simulink model "correlator_core"  (Simulink 7.1)
settings: Solver=ode45  StartTime=0.0  StopTime=10000  RelTol=1e-3
libraries: xbsIndex_r4 x658, cfa_library x168, casper_library_delays x4, casper_library_misc x2
(part 3 of 9)

== system correlator_core/correlator_core/ctrl ==
  integ_time : Inport
  Logical : xbsIndex_r4/Logical  logical_function=AND  inputs=2  en=off  latency=0  precision=Full  arith_type=Unsigned  n_bits=16  bin_pt=0  align_bp=on  dbl_ovrd=off  block_type=logical
      settings: block_version=11.4
  Relational : xbsIndex_r4/Relational  mode=a=b  en=off  latency=1  dbl_ovrd=off  block_type=relational
  frame_cntr : xbsIndex_r4/Counter  cnt_type=Free Running  cnt_to=Inf  operation=Up  start_count=0  cnt_by_val=1  arith_type=Unsigned  n_bits=32  bin_pt=0  load_pin=off  rst=on  en=on  explicit_period=on  period=1  dbl_ovrd=off  use_behavioral_HDL=off  use_rpm=off  implementation=Fabric  block_type=counter
      settings: block_version=11.4
  integ_cntr : xbsIndex_r4/Counter  cnt_type=Free Running  cnt_to=Inf  operation=Up  start_count=0  cnt_by_val=1  arith_type=Unsigned  n_bits=32  bin_pt=0  load_pin=off  rst=off  en=on  explicit_period=on  period=1  dbl_ovrd=off  use_behavioral_HDL=off  use_rpm=off  implementation=Fabric  block_type=counter
      settings: block_version=11.4
  lag_cntr : xbsIndex_r4/Counter  cnt_type=Free Running  cnt_to=Inf  operation=Up  start_count=0  cnt_by_val=1  arith_type=Unsigned  n_bits=5  bin_pt=0  load_pin=off  rst=on  en=off  explicit_period=on  period=1  dbl_ovrd=off  use_behavioral_HDL=off  use_rpm=off  implementation=Fabric  block_type=counter
      settings: block_version=11.4
  posedge1 : casper_library_misc/posedge  Tag=Rising Edge Detector  SystemSampleTime=-1
  integs : Outport
  tag scope: frames=global, lags=global, new_acc=global
  wires:
  frame_cntr/1 -> Relational/2, [frames]
  Logical/1 -> frame_cntr/1
  Relational/1 -> posedge1/1
  posedge1/1 -> Logical/1, integ_cntr/1, [new_acc]
  integ_time/1 -> Relational/1
  integ_cntr/1 -> integs/1
  lag_cntr/1 -> [lags]
  [sync_out] -> Logical/2, lag_cntr/1
  [valid_out] -> frame_cntr/2

== system correlator_core/correlator_core/delay_wideband_prog ==
  sync : Inport
  delay : Inport  Port=2
  en : Inport  Port=3
  data_in1 : Inport  Port=4
  data_in2 : Inport  Port=5
  data_in3 : Inport  Port=6
  data_in4 : Inport  Port=7
  AddSub1 : xbsIndex_r4/AddSub  mode=Addition  use_carryin=off  use_carryout=off  en=off  latency=0  precision=Full  arith_type=Unsigned  n_bits=9  bin_pt=0  quantization=Truncate  overflow=Wrap  dbl_ovrd=off  use_behavioral_HDL=off  pipelined=off  use_rpm=on  hw_selection=Fabric  block_type=addsub
  AddSub2 : xbsIndex_r4/AddSub  mode=Addition  use_carryin=off  use_carryout=off  en=off  latency=0  precision=Full  arith_type=Unsigned  n_bits=9  bin_pt=0  quantization=Truncate  overflow=Wrap  dbl_ovrd=off  use_behavioral_HDL=off  pipelined=off  use_rpm=on  hw_selection=Fabric  block_type=addsub
  AddSub3 : xbsIndex_r4/AddSub  mode=Addition  use_carryin=off  use_carryout=off  en=off  latency=0  precision=Full  arith_type=Unsigned  n_bits=9  bin_pt=0  quantization=Truncate  overflow=Wrap  dbl_ovrd=off  use_behavioral_HDL=off  pipelined=off  use_rpm=on  hw_selection=Fabric  block_type=addsub
  Constant1 : xbsIndex_r4/Constant  arith_type=Unsigned  const=2  n_bits=2  bin_pt=0  explicit_period=on  period=1  equ=P=C  opselect=C  inp2=PCIN>>17  opr=+  inp1=P  carry=CIN  dbl_ovrd=off  block_type=constant
      settings: block_version=11.4
  Constant2 : xbsIndex_r4/Constant  arith_type=Unsigned  const=1  n_bits=2  bin_pt=0  explicit_period=on  period=1  equ=P=C  opselect=C  inp2=PCIN>>17  opr=+  inp1=P  carry=CIN  dbl_ovrd=off  block_type=constant
      settings: block_version=11.4
  Constant3 : xbsIndex_r4/Constant  arith_type=Unsigned  const=0  n_bits=2  bin_pt=0  explicit_period=on  period=1  equ=P=C  opselect=C  inp2=PCIN>>17  opr=+  inp1=P  carry=CIN  dbl_ovrd=off  block_type=constant
      settings: block_version=11.4
  Convert1 : xbsIndex_r4/Convert  arith_type=Unsigned  n_bits=1  bin_pt=0  quantization=Truncate  overflow=Wrap  latency=0  dbl_ovrd=off  pipeline=off  block_type=convert
      settings: block_version=11.4
  Convert2 : xbsIndex_r4/Convert  arith_type=Unsigned  n_bits=1  bin_pt=0  quantization=Truncate  overflow=Wrap  latency=0  dbl_ovrd=off  pipeline=off  block_type=convert
      settings: block_version=11.4
  Convert3 : xbsIndex_r4/Convert  arith_type=Unsigned  n_bits=1  bin_pt=0  quantization=Truncate  overflow=Wrap  latency=0  dbl_ovrd=off  pipeline=off  block_type=convert
      settings: block_version=11.4
  Relational1 : xbsIndex_r4/Relational  mode=a>b  en=off  latency=0  dbl_ovrd=off  block_type=relational
  Relational2 : xbsIndex_r4/Relational  mode=a>b  en=off  latency=0  dbl_ovrd=off  block_type=relational
  Relational3 : xbsIndex_r4/Relational  mode=a>b  en=off  latency=0  dbl_ovrd=off  block_type=relational
  barrel_switcher : Subsystem  AncestorBlock=casper_library_reorder/barrel_switcher  mask(barrel_switcher){n_inputs=2}
      mask prompts: n_inputs "Number of Inputs: (2^?)"
      mask help:
      | Shifts input to right by amount specified on sel,
      | wrapping around into higher order bits.
      mask init:
      | barrel_switcher_init(gcb,...
      |     'n_inputs', n_inputs);
      settings: AttributesFormatString=n_inputs=2
      mask Help: eval('xlWeb(''http://casper.berkeley.edu/wiki/Barrel_switcher'')')
  bram_rd_addrs : xbsIndex_r4/Slice  nbits=9  boolean_output=off  mode=Lower Bit Location + Width  bit1=0  base1=MSB of Input  bit0=2  base0=LSB of Input  dbl_ovrd=off  block_type=slice
  delay_dp : casper_library_delays/delay_bram_prog_dp  SystemSampleTime=-1  ram_bits=9  bram_latency=2
      link override wr_addr: cnt_type=Free Running  cnt_to=Inf  operation=Up  start_count=0  cnt_by_val=1  arith_type=Unsigned  n_bits=ram_bits  bin_pt=0  load_pin=off  rst=off  en=off  explicit_period=on  period=1  dbl_ovrd=off  use_behavioral_HDL=on  implementation=Fabric  use_rpm=on
      link override wr_addr: infoedit="Hardware notes: Free running counters are the least expensive in hardware.  A count limited counter is implemented by combining a counter with a comparator."  xl_area=[0, 0, 0, 0, 0, 0, 0]
  delay_dp1 : casper_library_delays/delay_bram_prog_dp  SystemSampleTime=-1  ram_bits=9  bram_latency=2
  delay_dp2 : casper_library_delays/delay_bram_prog_dp  SystemSampleTime=-1  ram_bits=9  bram_latency=2
  delay_dp3 : casper_library_delays/delay_bram_prog_dp  SystemSampleTime=-1  ram_bits=9  bram_latency=2
  delay_reg : xbsIndex_r4/Register  init=0  rst=off  en=on  dbl_ovrd=off  block_type=register
      settings: block_version=11.4
  delay_sel : xbsIndex_r4/Delay  en=off  latency=3  dbl_ovrd=off  reg_retiming=off  block_type=delay
      settings: block_version=11.4
  shift_sel : xbsIndex_r4/Slice  nbits=2  boolean_output=off  mode=Lower Bit Location + Width  bit1=0  base1=MSB of Input  bit0=0  base0=LSB of Input  dbl_ovrd=off  block_type=slice
  sync_delay : xbsIndex_r4/Delay  en=off  latency=3  dbl_ovrd=off  reg_retiming=off  block_type=delay
      settings: block_version=11.4
  sync_out : Outport
  data_out1 : Outport  Port=2
  data_out2 : Outport  Port=3
  data_out3 : Outport  Port=4
  data_out4 : Outport  Port=5
  wires:
  sync/1 -> sync_delay/1
  delay/1 -> delay_reg/1
  en/1 -> delay_reg/2
  delay_reg/1 -> bram_rd_addrs/1, shift_sel/1
  data_in1/1 -> delay_dp/1
  bram_rd_addrs/1 -> delay_dp/2, AddSub1/1, AddSub2/1, AddSub3/1
  sync_delay/1 -> barrel_switcher/2(sync_in)
  barrel_switcher/1(sync_out) -> sync_out/1
  barrel_switcher/5(Out4) -> data_out1/1
  delay_dp/1 -> barrel_switcher/6(In4)
  shift_sel/1 -> delay_sel/1, Relational1/1, Relational2/1, Relational3/1
  delay_sel/1 -> barrel_switcher/1(sel)
  Constant1/1 -> Relational1/2
  Relational1/1 -> Convert1/1
  Convert1/1 -> AddSub1/2
  AddSub1/1 -> delay_dp1/2
  data_in2/1 -> delay_dp1/1
  delay_dp1/1 -> barrel_switcher/5(In3)
  barrel_switcher/2(Out1) -> data_out4/1
  Constant2/1 -> Relational2/2
  Relational2/1 -> Convert2/1
  Convert2/1 -> AddSub2/2
  AddSub2/1 -> delay_dp2/2
  data_in3/1 -> delay_dp2/1
  delay_dp2/1 -> barrel_switcher/4(In2)
  barrel_switcher/3(Out2) -> data_out3/1
  Constant3/1 -> Relational3/2
  Relational3/1 -> Convert3/1
  Convert3/1 -> AddSub3/2
  AddSub3/1 -> delay_dp3/2
  data_in4/1 -> delay_dp3/1
  delay_dp3/1 -> barrel_switcher/3(In1)
  barrel_switcher/4(Out3) -> data_out2/1

== system correlator_core/correlator_core/simple_bram_vacc ==
  new_acc : Inport  OutDataType=sfix(16)  OutScaling=2^0
  din : Inport  Port=2  OutDataType=sfix(16)  OutScaling=2^0
  Adder : xbsIndex_r4/AddSub  mode=Addition  use_carryin=off  use_carryout=off  en=off  latency=add_latency  precision=User Defined  arith_type="Signed  (2's comp)"  n_bits=n_bits  bin_pt=bin_pt  quantization=Truncate  overflow=Wrap  dbl_ovrd=off  use_behavioral_HDL=off  pipelined=on  use_rpm=on  hw_selection=Fabric  block_type=addsub
      settings: xl_area=[0, 0, 0, 0, 0, 0, 0]  block_version=10.1.3
  Constant : xbsIndex_r4/Constant  arith_type=Signed (2's comp)  const=0  n_bits=n_bits  bin_pt=bin_pt  explicit_period=on  period=1  equ=P=C  opselect=C  inp2=PCIN>>17  opr=+  inp1=P  carry=CIN  dbl_ovrd=off  block_type=constant
  Mux : xbsIndex_r4/Mux  inputs=2  en=off  latency=0  precision=Full  arith_type="Signed  (2's comp)"  n_bits=8  bin_pt=2  quantization=Truncate  overflow=Wrap  dbl_ovrd=off  block_type=mux
      settings: xl_area=[0, 0, 0, 0, 0, 0, 0]
  delay_bram : Subsystem  mask(delay_bram){DelayLen=vec_len - add_latency, bram_latency=add_latency}
      mask prompts: DelayLen "Delay By:"; bram_latency "BRAM Latency"
      mask help: A delay block that uses BRAM for its storage.
      mask init:
      | if (DelayLen <= bram_latency)
      | 	error('delay value must be greater than BRAM Latency');
      | end
      | BitWidth = max(ceil(log2(DelayLen)), 2);
      mask Help: eval('xlWeb(''http://casper.berkeley.edu/wiki/Delay_bram'')')
  pulse_ext : Subsystem  mask(pulse_ext){pulse_len=vec_len}
      mask prompts: pulse_len "Length of Pulse"
      mask help:
      | Extends a boolean signal to be high for the specified number of clocks after
      | the last high input.
      mask init:
      | bits = ceil(log2(pulse_len+1));
      mask Help: eval('xlWeb(''http://casper.berkeley.edu/wiki/Pulse_ext'')')
  dout : Outport  OutDataType=sfix(16)  OutScaling=2^0
  valid : Outport  Port=2  OutDataType=sfix(16)  OutScaling=2^0
  wires:
  Adder/1 -> delay_bram/1(In1)
  delay_bram/1(Out1) -> dout/1, Mux/2
  new_acc/1 -> pulse_ext/1(in)
  din/1 -> Adder/1
  pulse_ext/1(out) -> Mux/1, valid/1
  Mux/1 -> Adder/2
  Constant/1 -> Mux/3

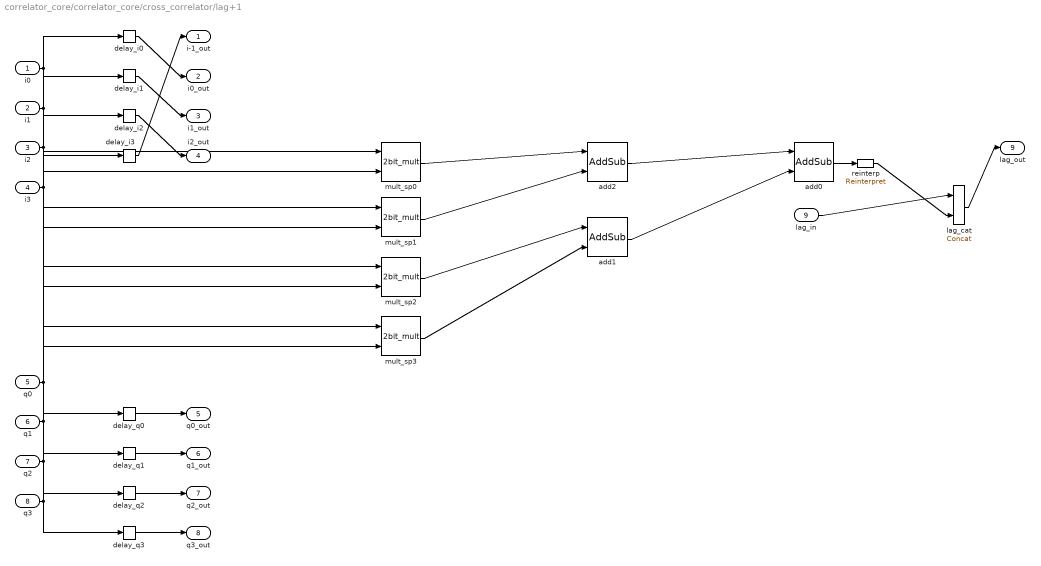
== system correlator_core/correlator_core/cross_correlator/lag+1 ==
  i0 : Inport
  i1 : Inport  Port=2
  i2 : Inport  Port=3
  i3 : Inport  Port=4
  q0 : Inport  Port=5
  q1 : Inport  Port=6
  q2 : Inport  Port=7
  q3 : Inport  Port=8
  lag_in : Inport  Port=9
  add0 : xbsIndex_r4/AddSub  mode=Addition  use_carryin=off  use_carryout=off  en=off  latency=2  precision=Full  arith_type=Unsigned  n_bits=16  bin_pt=14  quantization=Truncate  overflow=Wrap  dbl_ovrd=off  use_behavioral_HDL=on  pipelined=on  use_rpm=on  hw_selection=Fabric  block_type=addsub
  add1 : xbsIndex_r4/AddSub  mode=Addition  use_carryin=off  use_carryout=off  en=off  latency=2  precision=Full  arith_type=Unsigned  n_bits=16  bin_pt=14  quantization=Truncate  overflow=Wrap  dbl_ovrd=off  use_behavioral_HDL=on  pipelined=on  use_rpm=on  hw_selection=Fabric  block_type=addsub
      settings: block_version=10.1.3
  add2 : xbsIndex_r4/AddSub  mode=Addition  use_carryin=off  use_carryout=off  en=off  latency=2  precision=Full  arith_type=Unsigned  n_bits=16  bin_pt=14  quantization=Truncate  overflow=Wrap  dbl_ovrd=off  use_behavioral_HDL=on  pipelined=on  use_rpm=on  hw_selection=Fabric  block_type=addsub
      settings: block_version=10.1.3
  delay_i0 : xbsIndex_r4/Delay  en=off  latency=2  dbl_ovrd=off  reg_retiming=off  block_type=delay
      settings: block_version=11.4
  delay_i1 : xbsIndex_r4/Delay  en=off  latency=2  dbl_ovrd=off  reg_retiming=off  block_type=delay
      settings: block_version=11.4
  delay_i2 : xbsIndex_r4/Delay  en=off  latency=2  dbl_ovrd=off  reg_retiming=off  block_type=delay
  delay_i3 : xbsIndex_r4/Delay  en=off  latency=3  dbl_ovrd=off  reg_retiming=off  block_type=delay
  delay_q{0..3} (4 alike) : xbsIndex_r4/Delay  en=off  latency=2  dbl_ovrd=off  reg_retiming=off  block_type=delay
      delay_q0 settings: block_version=11.4
      delay_q1 settings: block_version=11.4
  lag_cat : xbsIndex_r4/Concat  num_inputs=2  dbl_ovrd=off  block_type=concat
  mult_sp{0..3} (4 alike) : cfa_library/2bit_mult  SystemSampleTime=-1
  reinterp : xbsIndex_r4/Reinterpret  force_arith_type=on  arith_type=Unsigned  force_bin_pt=on  bin_pt=0  block_type=reinterpret
      settings: infoedit="Changes signal type without altering the binary representation.   You can changed the signal between signed and unsigned, and relocate the binary point.<br><br>Hardware notes: In hardware this block costs nothing.<br><br>Example:  Suppose the input is 6 bits wide, signed, with 2 fractional bits, and the output is forced to unsigned with 0 fractional bits.  Then an input of -2.0 (1110.00 in binary 2's complement) becomes an output of 56 (111000 in binary)."
  i-1_out : Outport
  i0_out : Outport  Port=2
  i1_out : Outport  Port=3
  i2_out : Outport  Port=4
  q0_out : Outport  Port=5
  q1_out : Outport  Port=6
  q2_out : Outport  Port=7
  q3_out : Outport  Port=8
  lag_out : Outport  Port=9
  wires:
  i0/1 -> mult_sp0/1, delay_i0/1
  q0/1 -> mult_sp0/2, delay_q0/1
  i1/1 -> mult_sp1/1, delay_i1/1
  q1/1 -> mult_sp1/2, delay_q1/1
  i2/1 -> mult_sp2/1, delay_i2/1
  q2/1 -> mult_sp2/2, delay_q2/1
  i3/1 -> mult_sp3/1, delay_i3/1
  q3/1 -> mult_sp3/2, delay_q3/1
  mult_sp0/1 -> add2/1
  mult_sp1/1 -> add2/2
  mult_sp2/1 -> add1/1
  mult_sp3/1 -> add1/2
  add2/1 -> add0/1
  add1/1 -> add0/2
  delay_i0/1 -> i0_out/1
  delay_q0/1 -> q0_out/1
  delay_i1/1 -> i1_out/1
  delay_q1/1 -> q1_out/1
  delay_i2/1 -> i2_out/1
  delay_q2/1 -> q2_out/1
  delay_i3/1 -> i-1_out/1
  delay_q3/1 -> q3_out/1
  lag_in/1 -> lag_cat/1
  add0/1 -> reinterp/1
  reinterp/1 -> lag_cat/2
  lag_cat/1 -> lag_out/1

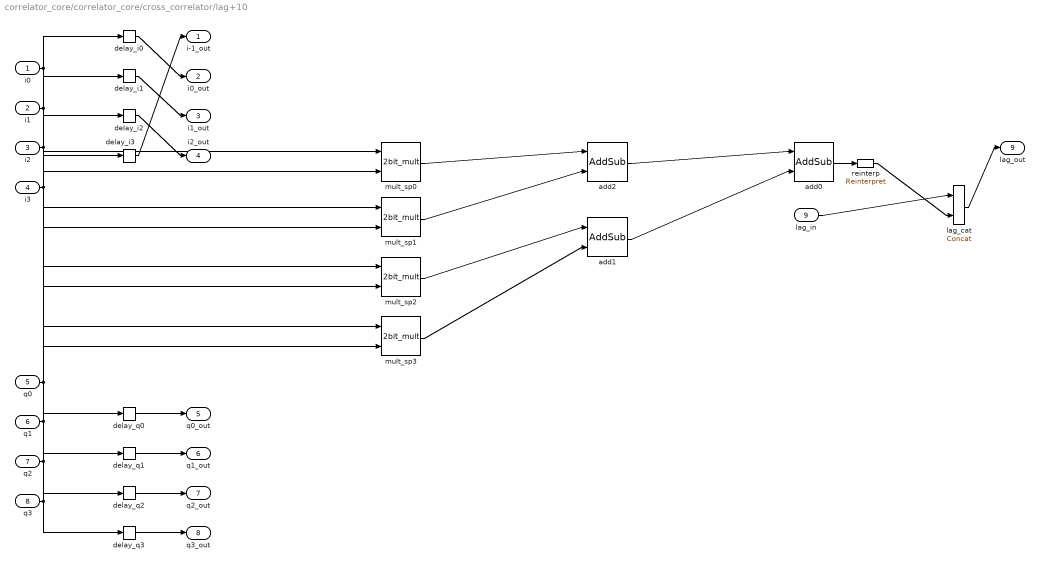
== system correlator_core/correlator_core/cross_correlator/lag+10 ==
  i0 : Inport
  i1 : Inport  Port=2
  i2 : Inport  Port=3
  i3 : Inport  Port=4
  q0 : Inport  Port=5
  q1 : Inport  Port=6
  q2 : Inport  Port=7
  q3 : Inport  Port=8
  lag_in : Inport  Port=9
  add0 : xbsIndex_r4/AddSub  mode=Addition  use_carryin=off  use_carryout=off  en=off  latency=2  precision=Full  arith_type=Unsigned  n_bits=16  bin_pt=14  quantization=Truncate  overflow=Wrap  dbl_ovrd=off  use_behavioral_HDL=on  pipelined=on  use_rpm=on  hw_selection=Fabric  block_type=addsub
  add1 : xbsIndex_r4/AddSub  mode=Addition  use_carryin=off  use_carryout=off  en=off  latency=2  precision=Full  arith_type=Unsigned  n_bits=16  bin_pt=14  quantization=Truncate  overflow=Wrap  dbl_ovrd=off  use_behavioral_HDL=on  pipelined=on  use_rpm=on  hw_selection=Fabric  block_type=addsub
      settings: block_version=10.1.3
  add2 : xbsIndex_r4/AddSub  mode=Addition  use_carryin=off  use_carryout=off  en=off  latency=2  precision=Full  arith_type=Unsigned  n_bits=16  bin_pt=14  quantization=Truncate  overflow=Wrap  dbl_ovrd=off  use_behavioral_HDL=on  pipelined=on  use_rpm=on  hw_selection=Fabric  block_type=addsub
      settings: block_version=10.1.3
  delay_i0 : xbsIndex_r4/Delay  en=off  latency=2  dbl_ovrd=off  reg_retiming=off  block_type=delay
      settings: block_version=11.4
  delay_i1 : xbsIndex_r4/Delay  en=off  latency=2  dbl_ovrd=off  reg_retiming=off  block_type=delay
      settings: block_version=11.4
  delay_i2 : xbsIndex_r4/Delay  en=off  latency=2  dbl_ovrd=off  reg_retiming=off  block_type=delay
  delay_i3 : xbsIndex_r4/Delay  en=off  latency=3  dbl_ovrd=off  reg_retiming=off  block_type=delay
  delay_q{0..3} (4 alike) : xbsIndex_r4/Delay  en=off  latency=2  dbl_ovrd=off  reg_retiming=off  block_type=delay
      delay_q0 settings: block_version=11.4
      delay_q1 settings: block_version=11.4
  lag_cat : xbsIndex_r4/Concat  num_inputs=2  dbl_ovrd=off  block_type=concat
  mult_sp{0..3} (4 alike) : cfa_library/2bit_mult  SystemSampleTime=-1
  reinterp : xbsIndex_r4/Reinterpret  force_arith_type=on  arith_type=Unsigned  force_bin_pt=on  bin_pt=0  block_type=reinterpret
      settings: infoedit="Changes signal type without altering the binary representation.   You can changed the signal between signed and unsigned, and relocate the binary point.<br><br>Hardware notes: In hardware this block costs nothing.<br><br>Example:  Suppose the input is 6 bits wide, signed, with 2 fractional bits, and the output is forced to unsigned with 0 fractional bits.  Then an input of -2.0 (1110.00 in binary 2's complement) becomes an output of 56 (111000 in binary)."
  i-1_out : Outport
  i0_out : Outport  Port=2
  i1_out : Outport  Port=3
  i2_out : Outport  Port=4
  q0_out : Outport  Port=5
  q1_out : Outport  Port=6
  q2_out : Outport  Port=7
  q3_out : Outport  Port=8
  lag_out : Outport  Port=9
  wires:
  i0/1 -> mult_sp0/1, delay_i0/1
  q0/1 -> mult_sp0/2, delay_q0/1
  i1/1 -> mult_sp1/1, delay_i1/1
  q1/1 -> mult_sp1/2, delay_q1/1
  i2/1 -> mult_sp2/1, delay_i2/1
  q2/1 -> mult_sp2/2, delay_q2/1
  i3/1 -> mult_sp3/1, delay_i3/1
  q3/1 -> mult_sp3/2, delay_q3/1
  mult_sp0/1 -> add2/1
  mult_sp1/1 -> add2/2
  mult_sp2/1 -> add1/1
  mult_sp3/1 -> add1/2
  add2/1 -> add0/1
  add1/1 -> add0/2
  delay_i0/1 -> i0_out/1
  delay_q0/1 -> q0_out/1
  delay_i1/1 -> i1_out/1
  delay_q1/1 -> q1_out/1
  delay_i2/1 -> i2_out/1
  delay_q2/1 -> q2_out/1
  delay_i3/1 -> i-1_out/1
  delay_q3/1 -> q3_out/1
  lag_in/1 -> lag_cat/1
  add0/1 -> reinterp/1
  reinterp/1 -> lag_cat/2
  lag_cat/1 -> lag_out/1

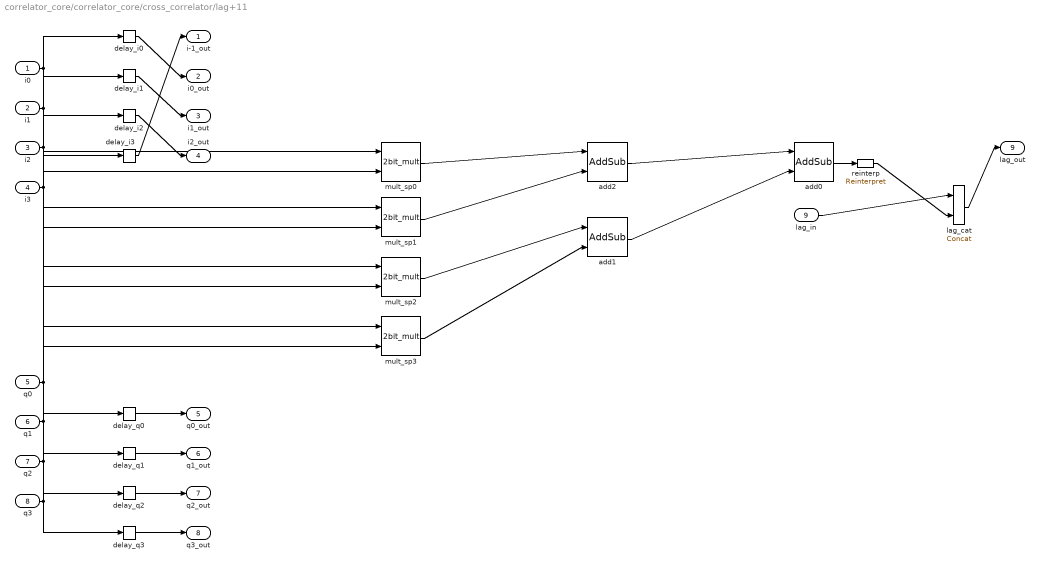
== system correlator_core/correlator_core/cross_correlator/lag+11 ==
  i0 : Inport
  i1 : Inport  Port=2
  i2 : Inport  Port=3
  i3 : Inport  Port=4
  q0 : Inport  Port=5
  q1 : Inport  Port=6
  q2 : Inport  Port=7
  q3 : Inport  Port=8
  lag_in : Inport  Port=9
  add0 : xbsIndex_r4/AddSub  mode=Addition  use_carryin=off  use_carryout=off  en=off  latency=2  precision=Full  arith_type=Unsigned  n_bits=16  bin_pt=14  quantization=Truncate  overflow=Wrap  dbl_ovrd=off  use_behavioral_HDL=on  pipelined=on  use_rpm=on  hw_selection=Fabric  block_type=addsub
  add1 : xbsIndex_r4/AddSub  mode=Addition  use_carryin=off  use_carryout=off  en=off  latency=2  precision=Full  arith_type=Unsigned  n_bits=16  bin_pt=14  quantization=Truncate  overflow=Wrap  dbl_ovrd=off  use_behavioral_HDL=on  pipelined=on  use_rpm=on  hw_selection=Fabric  block_type=addsub
      settings: block_version=10.1.3
  add2 : xbsIndex_r4/AddSub  mode=Addition  use_carryin=off  use_carryout=off  en=off  latency=2  precision=Full  arith_type=Unsigned  n_bits=16  bin_pt=14  quantization=Truncate  overflow=Wrap  dbl_ovrd=off  use_behavioral_HDL=on  pipelined=on  use_rpm=on  hw_selection=Fabric  block_type=addsub
      settings: block_version=10.1.3
  delay_i0 : xbsIndex_r4/Delay  en=off  latency=2  dbl_ovrd=off  reg_retiming=off  block_type=delay
      settings: block_version=11.4
  delay_i1 : xbsIndex_r4/Delay  en=off  latency=2  dbl_ovrd=off  reg_retiming=off  block_type=delay
      settings: block_version=11.4
  delay_i2 : xbsIndex_r4/Delay  en=off  latency=2  dbl_ovrd=off  reg_retiming=off  block_type=delay
  delay_i3 : xbsIndex_r4/Delay  en=off  latency=3  dbl_ovrd=off  reg_retiming=off  block_type=delay
  delay_q{0..3} (4 alike) : xbsIndex_r4/Delay  en=off  latency=2  dbl_ovrd=off  reg_retiming=off  block_type=delay
      delay_q0 settings: block_version=11.4
      delay_q1 settings: block_version=11.4
  lag_cat : xbsIndex_r4/Concat  num_inputs=2  dbl_ovrd=off  block_type=concat
  mult_sp{0..3} (4 alike) : cfa_library/2bit_mult  SystemSampleTime=-1
  reinterp : xbsIndex_r4/Reinterpret  force_arith_type=on  arith_type=Unsigned  force_bin_pt=on  bin_pt=0  block_type=reinterpret
      settings: infoedit="Changes signal type without altering the binary representation.   You can changed the signal between signed and unsigned, and relocate the binary point.<br><br>Hardware notes: In hardware this block costs nothing.<br><br>Example:  Suppose the input is 6 bits wide, signed, with 2 fractional bits, and the output is forced to unsigned with 0 fractional bits.  Then an input of -2.0 (1110.00 in binary 2's complement) becomes an output of 56 (111000 in binary)."
  i-1_out : Outport
  i0_out : Outport  Port=2
  i1_out : Outport  Port=3
  i2_out : Outport  Port=4
  q0_out : Outport  Port=5
  q1_out : Outport  Port=6
  q2_out : Outport  Port=7
  q3_out : Outport  Port=8
  lag_out : Outport  Port=9
  wires:
  i0/1 -> mult_sp0/1, delay_i0/1
  q0/1 -> mult_sp0/2, delay_q0/1
  i1/1 -> mult_sp1/1, delay_i1/1
  q1/1 -> mult_sp1/2, delay_q1/1
  i2/1 -> mult_sp2/1, delay_i2/1
  q2/1 -> mult_sp2/2, delay_q2/1
  i3/1 -> mult_sp3/1, delay_i3/1
  q3/1 -> mult_sp3/2, delay_q3/1
  mult_sp0/1 -> add2/1
  mult_sp1/1 -> add2/2
  mult_sp2/1 -> add1/1
  mult_sp3/1 -> add1/2
  add2/1 -> add0/1
  add1/1 -> add0/2
  delay_i0/1 -> i0_out/1
  delay_q0/1 -> q0_out/1
  delay_i1/1 -> i1_out/1
  delay_q1/1 -> q1_out/1
  delay_i2/1 -> i2_out/1
  delay_q2/1 -> q2_out/1
  delay_i3/1 -> i-1_out/1
  delay_q3/1 -> q3_out/1
  lag_in/1 -> lag_cat/1
  add0/1 -> reinterp/1
  reinterp/1 -> lag_cat/2
  lag_cat/1 -> lag_out/1

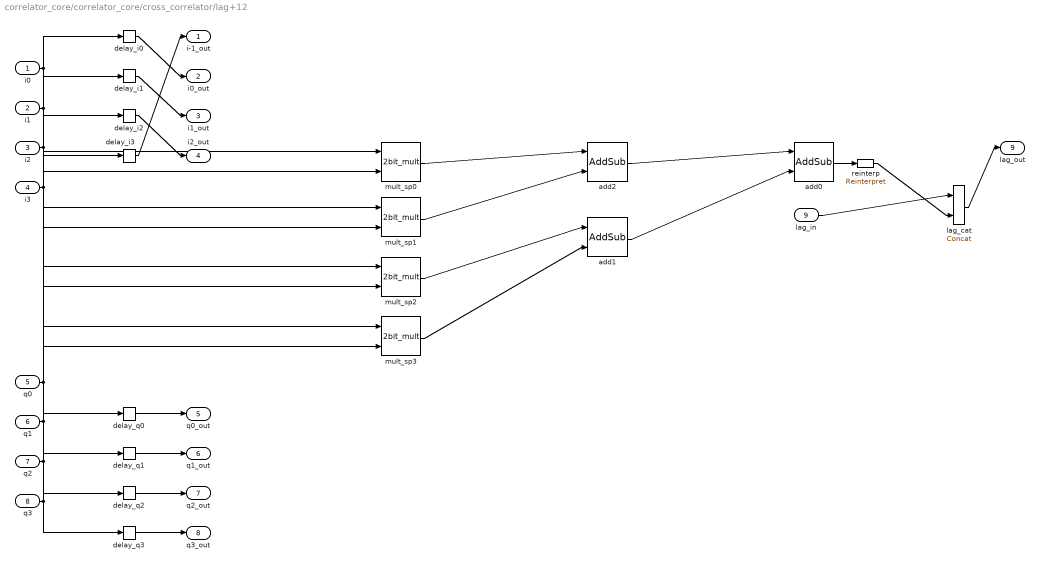
== system correlator_core/correlator_core/cross_correlator/lag+12 ==
  i0 : Inport
  i1 : Inport  Port=2
  i2 : Inport  Port=3
  i3 : Inport  Port=4
  q0 : Inport  Port=5
  q1 : Inport  Port=6
  q2 : Inport  Port=7
  q3 : Inport  Port=8
  lag_in : Inport  Port=9
  add0 : xbsIndex_r4/AddSub  mode=Addition  use_carryin=off  use_carryout=off  en=off  latency=2  precision=Full  arith_type=Unsigned  n_bits=16  bin_pt=14  quantization=Truncate  overflow=Wrap  dbl_ovrd=off  use_behavioral_HDL=on  pipelined=on  use_rpm=on  hw_selection=Fabric  block_type=addsub
  add1 : xbsIndex_r4/AddSub  mode=Addition  use_carryin=off  use_carryout=off  en=off  latency=2  precision=Full  arith_type=Unsigned  n_bits=16  bin_pt=14  quantization=Truncate  overflow=Wrap  dbl_ovrd=off  use_behavioral_HDL=on  pipelined=on  use_rpm=on  hw_selection=Fabric  block_type=addsub
      settings: block_version=10.1.3
  add2 : xbsIndex_r4/AddSub  mode=Addition  use_carryin=off  use_carryout=off  en=off  latency=2  precision=Full  arith_type=Unsigned  n_bits=16  bin_pt=14  quantization=Truncate  overflow=Wrap  dbl_ovrd=off  use_behavioral_HDL=on  pipelined=on  use_rpm=on  hw_selection=Fabric  block_type=addsub
      settings: block_version=10.1.3
  delay_i0 : xbsIndex_r4/Delay  en=off  latency=2  dbl_ovrd=off  reg_retiming=off  block_type=delay
      settings: block_version=11.4
  delay_i1 : xbsIndex_r4/Delay  en=off  latency=2  dbl_ovrd=off  reg_retiming=off  block_type=delay
      settings: block_version=11.4
  delay_i2 : xbsIndex_r4/Delay  en=off  latency=2  dbl_ovrd=off  reg_retiming=off  block_type=delay
  delay_i3 : xbsIndex_r4/Delay  en=off  latency=3  dbl_ovrd=off  reg_retiming=off  block_type=delay
  delay_q{0..3} (4 alike) : xbsIndex_r4/Delay  en=off  latency=2  dbl_ovrd=off  reg_retiming=off  block_type=delay
      delay_q0 settings: block_version=11.4
      delay_q1 settings: block_version=11.4
  lag_cat : xbsIndex_r4/Concat  num_inputs=2  dbl_ovrd=off  block_type=concat
  mult_sp{0..3} (4 alike) : cfa_library/2bit_mult  SystemSampleTime=-1
  reinterp : xbsIndex_r4/Reinterpret  force_arith_type=on  arith_type=Unsigned  force_bin_pt=on  bin_pt=0  block_type=reinterpret
      settings: infoedit="Changes signal type without altering the binary representation.   You can changed the signal between signed and unsigned, and relocate the binary point.<br><br>Hardware notes: In hardware this block costs nothing.<br><br>Example:  Suppose the input is 6 bits wide, signed, with 2 fractional bits, and the output is forced to unsigned with 0 fractional bits.  Then an input of -2.0 (1110.00 in binary 2's complement) becomes an output of 56 (111000 in binary)."
  i-1_out : Outport
  i0_out : Outport  Port=2
  i1_out : Outport  Port=3
  i2_out : Outport  Port=4
  q0_out : Outport  Port=5
  q1_out : Outport  Port=6
  q2_out : Outport  Port=7
  q3_out : Outport  Port=8
  lag_out : Outport  Port=9
  wires:
  i0/1 -> mult_sp0/1, delay_i0/1
  q0/1 -> mult_sp0/2, delay_q0/1
  i1/1 -> mult_sp1/1, delay_i1/1
  q1/1 -> mult_sp1/2, delay_q1/1
  i2/1 -> mult_sp2/1, delay_i2/1
  q2/1 -> mult_sp2/2, delay_q2/1
  i3/1 -> mult_sp3/1, delay_i3/1
  q3/1 -> mult_sp3/2, delay_q3/1
  mult_sp0/1 -> add2/1
  mult_sp1/1 -> add2/2
  mult_sp2/1 -> add1/1
  mult_sp3/1 -> add1/2
  add2/1 -> add0/1
  add1/1 -> add0/2
  delay_i0/1 -> i0_out/1
  delay_q0/1 -> q0_out/1
  delay_i1/1 -> i1_out/1
  delay_q1/1 -> q1_out/1
  delay_i2/1 -> i2_out/1
  delay_q2/1 -> q2_out/1
  delay_i3/1 -> i-1_out/1
  delay_q3/1 -> q3_out/1
  lag_in/1 -> lag_cat/1
  add0/1 -> reinterp/1
  reinterp/1 -> lag_cat/2
  lag_cat/1 -> lag_out/1

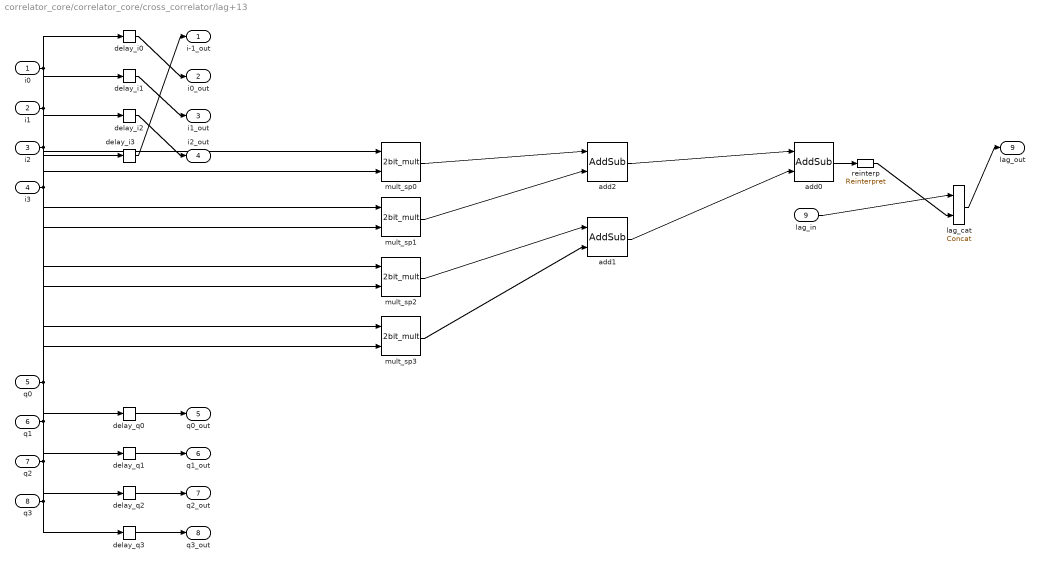
== system correlator_core/correlator_core/cross_correlator/lag+13 ==
  i0 : Inport
  i1 : Inport  Port=2
  i2 : Inport  Port=3
  i3 : Inport  Port=4
  q0 : Inport  Port=5
  q1 : Inport  Port=6
  q2 : Inport  Port=7
  q3 : Inport  Port=8
  lag_in : Inport  Port=9
  add0 : xbsIndex_r4/AddSub  mode=Addition  use_carryin=off  use_carryout=off  en=off  latency=2  precision=Full  arith_type=Unsigned  n_bits=16  bin_pt=14  quantization=Truncate  overflow=Wrap  dbl_ovrd=off  use_behavioral_HDL=on  pipelined=on  use_rpm=on  hw_selection=Fabric  block_type=addsub
  add1 : xbsIndex_r4/AddSub  mode=Addition  use_carryin=off  use_carryout=off  en=off  latency=2  precision=Full  arith_type=Unsigned  n_bits=16  bin_pt=14  quantization=Truncate  overflow=Wrap  dbl_ovrd=off  use_behavioral_HDL=on  pipelined=on  use_rpm=on  hw_selection=Fabric  block_type=addsub
      settings: block_version=10.1.3
  add2 : xbsIndex_r4/AddSub  mode=Addition  use_carryin=off  use_carryout=off  en=off  latency=2  precision=Full  arith_type=Unsigned  n_bits=16  bin_pt=14  quantization=Truncate  overflow=Wrap  dbl_ovrd=off  use_behavioral_HDL=on  pipelined=on  use_rpm=on  hw_selection=Fabric  block_type=addsub
      settings: block_version=10.1.3
  delay_i0 : xbsIndex_r4/Delay  en=off  latency=2  dbl_ovrd=off  reg_retiming=off  block_type=delay
      settings: block_version=11.4
  delay_i1 : xbsIndex_r4/Delay  en=off  latency=2  dbl_ovrd=off  reg_retiming=off  block_type=delay
      settings: block_version=11.4
  delay_i2 : xbsIndex_r4/Delay  en=off  latency=2  dbl_ovrd=off  reg_retiming=off  block_type=delay
  delay_i3 : xbsIndex_r4/Delay  en=off  latency=3  dbl_ovrd=off  reg_retiming=off  block_type=delay
  delay_q{0..3} (4 alike) : xbsIndex_r4/Delay  en=off  latency=2  dbl_ovrd=off  reg_retiming=off  block_type=delay
      delay_q0 settings: block_version=11.4
      delay_q1 settings: block_version=11.4
  lag_cat : xbsIndex_r4/Concat  num_inputs=2  dbl_ovrd=off  block_type=concat
  mult_sp{0..3} (4 alike) : cfa_library/2bit_mult  SystemSampleTime=-1
  reinterp : xbsIndex_r4/Reinterpret  force_arith_type=on  arith_type=Unsigned  force_bin_pt=on  bin_pt=0  block_type=reinterpret
      settings: infoedit="Changes signal type without altering the binary representation.   You can changed the signal between signed and unsigned, and relocate the binary point.<br><br>Hardware notes: In hardware this block costs nothing.<br><br>Example:  Suppose the input is 6 bits wide, signed, with 2 fractional bits, and the output is forced to unsigned with 0 fractional bits.  Then an input of -2.0 (1110.00 in binary 2's complement) becomes an output of 56 (111000 in binary)."
  i-1_out : Outport
  i0_out : Outport  Port=2
  i1_out : Outport  Port=3
  i2_out : Outport  Port=4
  q0_out : Outport  Port=5
  q1_out : Outport  Port=6
  q2_out : Outport  Port=7
  q3_out : Outport  Port=8
  lag_out : Outport  Port=9
  wires:
  i0/1 -> mult_sp0/1, delay_i0/1
  q0/1 -> mult_sp0/2, delay_q0/1
  i1/1 -> mult_sp1/1, delay_i1/1
  q1/1 -> mult_sp1/2, delay_q1/1
  i2/1 -> mult_sp2/1, delay_i2/1
  q2/1 -> mult_sp2/2, delay_q2/1
  i3/1 -> mult_sp3/1, delay_i3/1
  q3/1 -> mult_sp3/2, delay_q3/1
  mult_sp0/1 -> add2/1
  mult_sp1/1 -> add2/2
  mult_sp2/1 -> add1/1
  mult_sp3/1 -> add1/2
  add2/1 -> add0/1
  add1/1 -> add0/2
  delay_i0/1 -> i0_out/1
  delay_q0/1 -> q0_out/1
  delay_i1/1 -> i1_out/1
  delay_q1/1 -> q1_out/1
  delay_i2/1 -> i2_out/1
  delay_q2/1 -> q2_out/1
  delay_i3/1 -> i-1_out/1
  delay_q3/1 -> q3_out/1
  lag_in/1 -> lag_cat/1
  add0/1 -> reinterp/1
  reinterp/1 -> lag_cat/2
  lag_cat/1 -> lag_out/1

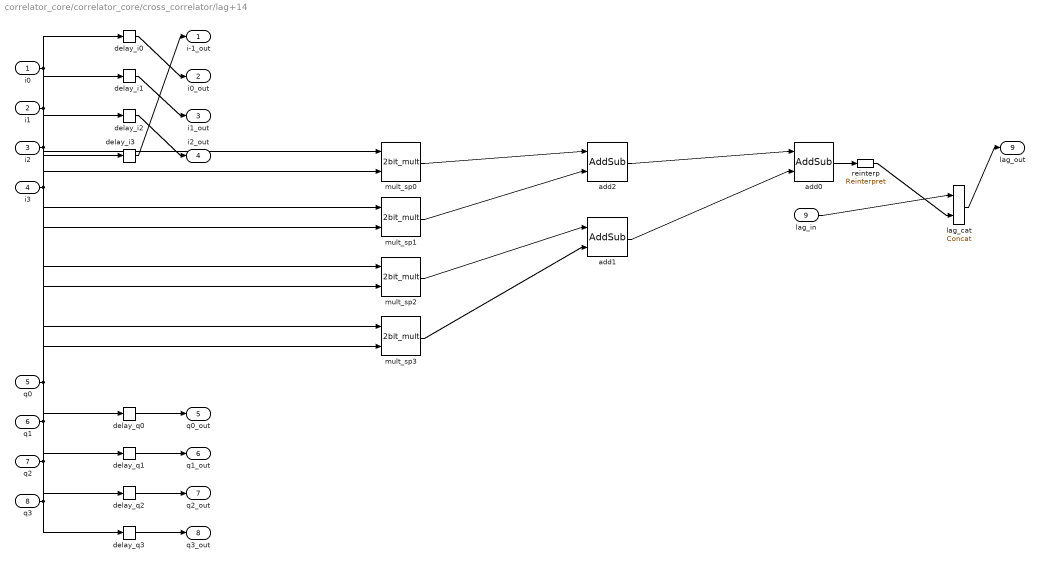
== system correlator_core/correlator_core/cross_correlator/lag+14 ==
  i0 : Inport
  i1 : Inport  Port=2
  i2 : Inport  Port=3
  i3 : Inport  Port=4
  q0 : Inport  Port=5
  q1 : Inport  Port=6
  q2 : Inport  Port=7
  q3 : Inport  Port=8
  lag_in : Inport  Port=9
  add0 : xbsIndex_r4/AddSub  mode=Addition  use_carryin=off  use_carryout=off  en=off  latency=2  precision=Full  arith_type=Unsigned  n_bits=16  bin_pt=14  quantization=Truncate  overflow=Wrap  dbl_ovrd=off  use_behavioral_HDL=on  pipelined=on  use_rpm=on  hw_selection=Fabric  block_type=addsub
  add1 : xbsIndex_r4/AddSub  mode=Addition  use_carryin=off  use_carryout=off  en=off  latency=2  precision=Full  arith_type=Unsigned  n_bits=16  bin_pt=14  quantization=Truncate  overflow=Wrap  dbl_ovrd=off  use_behavioral_HDL=on  pipelined=on  use_rpm=on  hw_selection=Fabric  block_type=addsub
      settings: block_version=10.1.3
  add2 : xbsIndex_r4/AddSub  mode=Addition  use_carryin=off  use_carryout=off  en=off  latency=2  precision=Full  arith_type=Unsigned  n_bits=16  bin_pt=14  quantization=Truncate  overflow=Wrap  dbl_ovrd=off  use_behavioral_HDL=on  pipelined=on  use_rpm=on  hw_selection=Fabric  block_type=addsub
      settings: block_version=10.1.3
  delay_i0 : xbsIndex_r4/Delay  en=off  latency=2  dbl_ovrd=off  reg_retiming=off  block_type=delay
      settings: block_version=11.4
  delay_i1 : xbsIndex_r4/Delay  en=off  latency=2  dbl_ovrd=off  reg_retiming=off  block_type=delay
      settings: block_version=11.4
  delay_i2 : xbsIndex_r4/Delay  en=off  latency=2  dbl_ovrd=off  reg_retiming=off  block_type=delay
  delay_i3 : xbsIndex_r4/Delay  en=off  latency=3  dbl_ovrd=off  reg_retiming=off  block_type=delay
  delay_q{0..3} (4 alike) : xbsIndex_r4/Delay  en=off  latency=2  dbl_ovrd=off  reg_retiming=off  block_type=delay
      delay_q0 settings: block_version=11.4
      delay_q1 settings: block_version=11.4
  lag_cat : xbsIndex_r4/Concat  num_inputs=2  dbl_ovrd=off  block_type=concat
  mult_sp{0..3} (4 alike) : cfa_library/2bit_mult  SystemSampleTime=-1
  reinterp : xbsIndex_r4/Reinterpret  force_arith_type=on  arith_type=Unsigned  force_bin_pt=on  bin_pt=0  block_type=reinterpret
      settings: infoedit="Changes signal type without altering the binary representation.   You can changed the signal between signed and unsigned, and relocate the binary point.<br><br>Hardware notes: In hardware this block costs nothing.<br><br>Example:  Suppose the input is 6 bits wide, signed, with 2 fractional bits, and the output is forced to unsigned with 0 fractional bits.  Then an input of -2.0 (1110.00 in binary 2's complement) becomes an output of 56 (111000 in binary)."
  i-1_out : Outport
  i0_out : Outport  Port=2
  i1_out : Outport  Port=3
  i2_out : Outport  Port=4
  q0_out : Outport  Port=5
  q1_out : Outport  Port=6
  q2_out : Outport  Port=7
  q3_out : Outport  Port=8
  lag_out : Outport  Port=9
  wires:
  i0/1 -> mult_sp0/1, delay_i0/1
  q0/1 -> mult_sp0/2, delay_q0/1
  i1/1 -> mult_sp1/1, delay_i1/1
  q1/1 -> mult_sp1/2, delay_q1/1
  i2/1 -> mult_sp2/1, delay_i2/1
  q2/1 -> mult_sp2/2, delay_q2/1
  i3/1 -> mult_sp3/1, delay_i3/1
  q3/1 -> mult_sp3/2, delay_q3/1
  mult_sp0/1 -> add2/1
  mult_sp1/1 -> add2/2
  mult_sp2/1 -> add1/1
  mult_sp3/1 -> add1/2
  add2/1 -> add0/1
  add1/1 -> add0/2
  delay_i0/1 -> i0_out/1
  delay_q0/1 -> q0_out/1
  delay_i1/1 -> i1_out/1
  delay_q1/1 -> q1_out/1
  delay_i2/1 -> i2_out/1
  delay_q2/1 -> q2_out/1
  delay_i3/1 -> i-1_out/1
  delay_q3/1 -> q3_out/1
  lag_in/1 -> lag_cat/1
  add0/1 -> reinterp/1
  reinterp/1 -> lag_cat/2
  lag_cat/1 -> lag_out/1

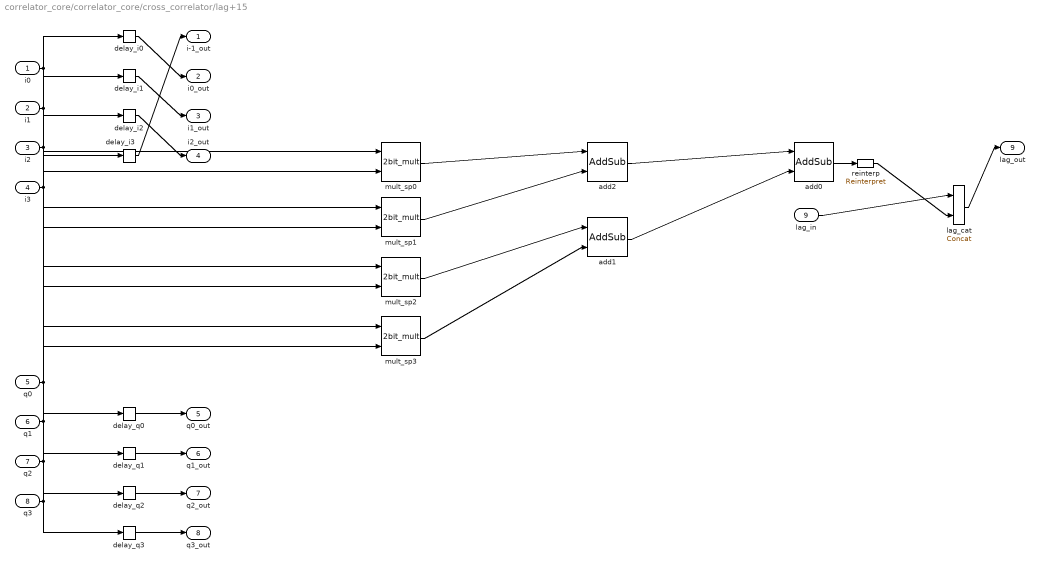
== system correlator_core/correlator_core/cross_correlator/lag+15 ==
  i0 : Inport
  i1 : Inport  Port=2
  i2 : Inport  Port=3
  i3 : Inport  Port=4
  q0 : Inport  Port=5
  q1 : Inport  Port=6
  q2 : Inport  Port=7
  q3 : Inport  Port=8
  lag_in : Inport  Port=9
  add0 : xbsIndex_r4/AddSub  mode=Addition  use_carryin=off  use_carryout=off  en=off  latency=2  precision=Full  arith_type=Unsigned  n_bits=16  bin_pt=14  quantization=Truncate  overflow=Wrap  dbl_ovrd=off  use_behavioral_HDL=on  pipelined=on  use_rpm=on  hw_selection=Fabric  block_type=addsub
  add1 : xbsIndex_r4/AddSub  mode=Addition  use_carryin=off  use_carryout=off  en=off  latency=2  precision=Full  arith_type=Unsigned  n_bits=16  bin_pt=14  quantization=Truncate  overflow=Wrap  dbl_ovrd=off  use_behavioral_HDL=on  pipelined=on  use_rpm=on  hw_selection=Fabric  block_type=addsub
      settings: block_version=10.1.3
  add2 : xbsIndex_r4/AddSub  mode=Addition  use_carryin=off  use_carryout=off  en=off  latency=2  precision=Full  arith_type=Unsigned  n_bits=16  bin_pt=14  quantization=Truncate  overflow=Wrap  dbl_ovrd=off  use_behavioral_HDL=on  pipelined=on  use_rpm=on  hw_selection=Fabric  block_type=addsub
      settings: block_version=10.1.3
  delay_i0 : xbsIndex_r4/Delay  en=off  latency=2  dbl_ovrd=off  reg_retiming=off  block_type=delay
      settings: block_version=11.4
  delay_i1 : xbsIndex_r4/Delay  en=off  latency=2  dbl_ovrd=off  reg_retiming=off  block_type=delay
      settings: block_version=11.4
  delay_i2 : xbsIndex_r4/Delay  en=off  latency=2  dbl_ovrd=off  reg_retiming=off  block_type=delay
  delay_i3 : xbsIndex_r4/Delay  en=off  latency=3  dbl_ovrd=off  reg_retiming=off  block_type=delay
  delay_q{0..3} (4 alike) : xbsIndex_r4/Delay  en=off  latency=2  dbl_ovrd=off  reg_retiming=off  block_type=delay
      delay_q0 settings: block_version=11.4
      delay_q1 settings: block_version=11.4
  lag_cat : xbsIndex_r4/Concat  num_inputs=2  dbl_ovrd=off  block_type=concat
  mult_sp{0..3} (4 alike) : cfa_library/2bit_mult  SystemSampleTime=-1
  reinterp : xbsIndex_r4/Reinterpret  force_arith_type=on  arith_type=Unsigned  force_bin_pt=on  bin_pt=0  block_type=reinterpret
      settings: infoedit="Changes signal type without altering the binary representation.   You can changed the signal between signed and unsigned, and relocate the binary point.<br><br>Hardware notes: In hardware this block costs nothing.<br><br>Example:  Suppose the input is 6 bits wide, signed, with 2 fractional bits, and the output is forced to unsigned with 0 fractional bits.  Then an input of -2.0 (1110.00 in binary 2's complement) becomes an output of 56 (111000 in binary)."
  i-1_out : Outport
  i0_out : Outport  Port=2
  i1_out : Outport  Port=3
  i2_out : Outport  Port=4
  q0_out : Outport  Port=5
  q1_out : Outport  Port=6
  q2_out : Outport  Port=7
  q3_out : Outport  Port=8
  lag_out : Outport  Port=9
  wires:
  i0/1 -> mult_sp0/1, delay_i0/1
  q0/1 -> mult_sp0/2, delay_q0/1
  i1/1 -> mult_sp1/1, delay_i1/1
  q1/1 -> mult_sp1/2, delay_q1/1
  i2/1 -> mult_sp2/1, delay_i2/1
  q2/1 -> mult_sp2/2, delay_q2/1
  i3/1 -> mult_sp3/1, delay_i3/1
  q3/1 -> mult_sp3/2, delay_q3/1
  mult_sp0/1 -> add2/1
  mult_sp1/1 -> add2/2
  mult_sp2/1 -> add1/1
  mult_sp3/1 -> add1/2
  add2/1 -> add0/1
  add1/1 -> add0/2
  delay_i0/1 -> i0_out/1
  delay_q0/1 -> q0_out/1
  delay_i1/1 -> i1_out/1
  delay_q1/1 -> q1_out/1
  delay_i2/1 -> i2_out/1
  delay_q2/1 -> q2_out/1
  delay_i3/1 -> i-1_out/1
  delay_q3/1 -> q3_out/1
  lag_in/1 -> lag_cat/1
  add0/1 -> reinterp/1
  reinterp/1 -> lag_cat/2
  lag_cat/1 -> lag_out/1

== system correlator_core/correlator_core/cross_correlator/lag+2 ==
  i0 : Inport
  i1 : Inport  Port=2
  i2 : Inport  Port=3
  i3 : Inport  Port=4
  q0 : Inport  Port=5
  q1 : Inport  Port=6
  q2 : Inport  Port=7
  q3 : Inport  Port=8
  lag_in : Inport  Port=9
  add0 : xbsIndex_r4/AddSub  mode=Addition  use_carryin=off  use_carryout=off  en=off  latency=2  precision=Full  arith_type=Unsigned  n_bits=16  bin_pt=14  quantization=Truncate  overflow=Wrap  dbl_ovrd=off  use_behavioral_HDL=on  pipelined=on  use_rpm=on  hw_selection=Fabric  block_type=addsub
  add1 : xbsIndex_r4/AddSub  mode=Addition  use_carryin=off  use_carryout=off  en=off  latency=2  precision=Full  arith_type=Unsigned  n_bits=16  bin_pt=14  quantization=Truncate  overflow=Wrap  dbl_ovrd=off  use_behavioral_HDL=on  pipelined=on  use_rpm=on  hw_selection=Fabric  block_type=addsub
      settings: block_version=10.1.3
  add2 : xbsIndex_r4/AddSub  mode=Addition  use_carryin=off  use_carryout=off  en=off  latency=2  precision=Full  arith_type=Unsigned  n_bits=16  bin_pt=14  quantization=Truncate  overflow=Wrap  dbl_ovrd=off  use_behavioral_HDL=on  pipelined=on  use_rpm=on  hw_selection=Fabric  block_type=addsub
      settings: block_version=10.1.3
  delay_i0 : xbsIndex_r4/Delay  en=off  latency=2  dbl_ovrd=off  reg_retiming=off  block_type=delay
      settings: block_version=11.4
  delay_i1 : xbsIndex_r4/Delay  en=off  latency=2  dbl_ovrd=off  reg_retiming=off  block_type=delay
      settings: block_version=11.4
  delay_i2 : xbsIndex_r4/Delay  en=off  latency=2  dbl_ovrd=off  reg_retiming=off  block_type=delay
  delay_i3 : xbsIndex_r4/Delay  en=off  latency=3  dbl_ovrd=off  reg_retiming=off  block_type=delay
  delay_q{0..3} (4 alike) : xbsIndex_r4/Delay  en=off  latency=2  dbl_ovrd=off  reg_retiming=off  block_type=delay
      delay_q0 settings: block_version=11.4
      delay_q1 settings: block_version=11.4
  lag_cat : xbsIndex_r4/Concat  num_inputs=2  dbl_ovrd=off  block_type=concat
  mult_sp{0..3} (4 alike) : cfa_library/2bit_mult  SystemSampleTime=-1
  reinterp : xbsIndex_r4/Reinterpret  force_arith_type=on  arith_type=Unsigned  force_bin_pt=on  bin_pt=0  block_type=reinterpret
      settings: infoedit="Changes signal type without altering the binary representation.   You can changed the signal between signed and unsigned, and relocate the binary point.<br><br>Hardware notes: In hardware this block costs nothing.<br><br>Example:  Suppose the input is 6 bits wide, signed, with 2 fractional bits, and the output is forced to unsigned with 0 fractional bits.  Then an input of -2.0 (1110.00 in binary 2's complement) becomes an output of 56 (111000 in binary)."
  i-1_out : Outport
  i0_out : Outport  Port=2
  i1_out : Outport  Port=3
  i2_out : Outport  Port=4
  q0_out : Outport  Port=5
  q1_out : Outport  Port=6
  q2_out : Outport  Port=7
  q3_out : Outport  Port=8
  lag_out : Outport  Port=9
  wires:
  i0/1 -> mult_sp0/1, delay_i0/1
  q0/1 -> mult_sp0/2, delay_q0/1
  i1/1 -> mult_sp1/1, delay_i1/1
  q1/1 -> mult_sp1/2, delay_q1/1
  i2/1 -> mult_sp2/1, delay_i2/1
  q2/1 -> mult_sp2/2, delay_q2/1
  i3/1 -> mult_sp3/1, delay_i3/1
  q3/1 -> mult_sp3/2, delay_q3/1
  mult_sp0/1 -> add2/1
  mult_sp1/1 -> add2/2
  mult_sp2/1 -> add1/1
  mult_sp3/1 -> add1/2
  add2/1 -> add0/1
  add1/1 -> add0/2
  delay_i0/1 -> i0_out/1
  delay_q0/1 -> q0_out/1
  delay_i1/1 -> i1_out/1
  delay_q1/1 -> q1_out/1
  delay_i2/1 -> i2_out/1
  delay_q2/1 -> q2_out/1
  delay_i3/1 -> i-1_out/1
  delay_q3/1 -> q3_out/1
  lag_in/1 -> lag_cat/1
  add0/1 -> reinterp/1
  reinterp/1 -> lag_cat/2
  lag_cat/1 -> lag_out/1

== system correlator_core/correlator_core/cross_correlator/lag+3 ==
  i0 : Inport
  i1 : Inport  Port=2
  i2 : Inport  Port=3
  i3 : Inport  Port=4
  q0 : Inport  Port=5
  q1 : Inport  Port=6
  q2 : Inport  Port=7
  q3 : Inport  Port=8
  lag_in : Inport  Port=9
  add0 : xbsIndex_r4/AddSub  mode=Addition  use_carryin=off  use_carryout=off  en=off  latency=2  precision=Full  arith_type=Unsigned  n_bits=16  bin_pt=14  quantization=Truncate  overflow=Wrap  dbl_ovrd=off  use_behavioral_HDL=on  pipelined=on  use_rpm=on  hw_selection=Fabric  block_type=addsub
  add1 : xbsIndex_r4/AddSub  mode=Addition  use_carryin=off  use_carryout=off  en=off  latency=2  precision=Full  arith_type=Unsigned  n_bits=16  bin_pt=14  quantization=Truncate  overflow=Wrap  dbl_ovrd=off  use_behavioral_HDL=on  pipelined=on  use_rpm=on  hw_selection=Fabric  block_type=addsub
      settings: block_version=10.1.3
  add2 : xbsIndex_r4/AddSub  mode=Addition  use_carryin=off  use_carryout=off  en=off  latency=2  precision=Full  arith_type=Unsigned  n_bits=16  bin_pt=14  quantization=Truncate  overflow=Wrap  dbl_ovrd=off  use_behavioral_HDL=on  pipelined=on  use_rpm=on  hw_selection=Fabric  block_type=addsub
      settings: block_version=10.1.3
  delay_i0 : xbsIndex_r4/Delay  en=off  latency=2  dbl_ovrd=off  reg_retiming=off  block_type=delay
      settings: block_version=11.4
  delay_i1 : xbsIndex_r4/Delay  en=off  latency=2  dbl_ovrd=off  reg_retiming=off  block_type=delay
      settings: block_version=11.4
  delay_i2 : xbsIndex_r4/Delay  en=off  latency=2  dbl_ovrd=off  reg_retiming=off  block_type=delay
  delay_i3 : xbsIndex_r4/Delay  en=off  latency=3  dbl_ovrd=off  reg_retiming=off  block_type=delay
  delay_q{0..3} (4 alike) : xbsIndex_r4/Delay  en=off  latency=2  dbl_ovrd=off  reg_retiming=off  block_type=delay
      delay_q0 settings: block_version=11.4
      delay_q1 settings: block_version=11.4
  lag_cat : xbsIndex_r4/Concat  num_inputs=2  dbl_ovrd=off  block_type=concat
  mult_sp{0..3} (4 alike) : cfa_library/2bit_mult  SystemSampleTime=-1
  reinterp : xbsIndex_r4/Reinterpret  force_arith_type=on  arith_type=Unsigned  force_bin_pt=on  bin_pt=0  block_type=reinterpret
      settings: infoedit="Changes signal type without altering the binary representation.   You can changed the signal between signed and unsigned, and relocate the binary point.<br><br>Hardware notes: In hardware this block costs nothing.<br><br>Example:  Suppose the input is 6 bits wide, signed, with 2 fractional bits, and the output is forced to unsigned with 0 fractional bits.  Then an input of -2.0 (1110.00 in binary 2's complement) becomes an output of 56 (111000 in binary)."
  i-1_out : Outport
  i0_out : Outport  Port=2
  i1_out : Outport  Port=3
  i2_out : Outport  Port=4
  q0_out : Outport  Port=5
  q1_out : Outport  Port=6
  q2_out : Outport  Port=7
  q3_out : Outport  Port=8
  lag_out : Outport  Port=9
  wires:
  i0/1 -> mult_sp0/1, delay_i0/1
  q0/1 -> mult_sp0/2, delay_q0/1
  i1/1 -> mult_sp1/1, delay_i1/1
  q1/1 -> mult_sp1/2, delay_q1/1
  i2/1 -> mult_sp2/1, delay_i2/1
  q2/1 -> mult_sp2/2, delay_q2/1
  i3/1 -> mult_sp3/1, delay_i3/1
  q3/1 -> mult_sp3/2, delay_q3/1
  mult_sp0/1 -> add2/1
  mult_sp1/1 -> add2/2
  mult_sp2/1 -> add1/1
  mult_sp3/1 -> add1/2
  add2/1 -> add0/1
  add1/1 -> add0/2
  delay_i0/1 -> i0_out/1
  delay_q0/1 -> q0_out/1
  delay_i1/1 -> i1_out/1
  delay_q1/1 -> q1_out/1
  delay_i2/1 -> i2_out/1
  delay_q2/1 -> q2_out/1
  delay_i3/1 -> i-1_out/1
  delay_q3/1 -> q3_out/1
  lag_in/1 -> lag_cat/1
  add0/1 -> reinterp/1
  reinterp/1 -> lag_cat/2
  lag_cat/1 -> lag_out/1

== system correlator_core/correlator_core/cross_correlator/lag+4 ==
  i0 : Inport
  i1 : Inport  Port=2
  i2 : Inport  Port=3
  i3 : Inport  Port=4
  q0 : Inport  Port=5
  q1 : Inport  Port=6
  q2 : Inport  Port=7
  q3 : Inport  Port=8
  lag_in : Inport  Port=9
  add0 : xbsIndex_r4/AddSub  mode=Addition  use_carryin=off  use_carryout=off  en=off  latency=2  precision=Full  arith_type=Unsigned  n_bits=16  bin_pt=14  quantization=Truncate  overflow=Wrap  dbl_ovrd=off  use_behavioral_HDL=on  pipelined=on  use_rpm=on  hw_selection=Fabric  block_type=addsub
  add1 : xbsIndex_r4/AddSub  mode=Addition  use_carryin=off  use_carryout=off  en=off  latency=2  precision=Full  arith_type=Unsigned  n_bits=16  bin_pt=14  quantization=Truncate  overflow=Wrap  dbl_ovrd=off  use_behavioral_HDL=on  pipelined=on  use_rpm=on  hw_selection=Fabric  block_type=addsub
      settings: block_version=10.1.3
  add2 : xbsIndex_r4/AddSub  mode=Addition  use_carryin=off  use_carryout=off  en=off  latency=2  precision=Full  arith_type=Unsigned  n_bits=16  bin_pt=14  quantization=Truncate  overflow=Wrap  dbl_ovrd=off  use_behavioral_HDL=on  pipelined=on  use_rpm=on  hw_selection=Fabric  block_type=addsub
      settings: block_version=10.1.3
  delay_i0 : xbsIndex_r4/Delay  en=off  latency=2  dbl_ovrd=off  reg_retiming=off  block_type=delay
      settings: block_version=11.4
  delay_i1 : xbsIndex_r4/Delay  en=off  latency=2  dbl_ovrd=off  reg_retiming=off  block_type=delay
      settings: block_version=11.4
  delay_i2 : xbsIndex_r4/Delay  en=off  latency=2  dbl_ovrd=off  reg_retiming=off  block_type=delay
  delay_i3 : xbsIndex_r4/Delay  en=off  latency=3  dbl_ovrd=off  reg_retiming=off  block_type=delay
  delay_q{0..3} (4 alike) : xbsIndex_r4/Delay  en=off  latency=2  dbl_ovrd=off  reg_retiming=off  block_type=delay
      delay_q0 settings: block_version=11.4
      delay_q1 settings: block_version=11.4
  lag_cat : xbsIndex_r4/Concat  num_inputs=2  dbl_ovrd=off  block_type=concat
  mult_sp{0..3} (4 alike) : cfa_library/2bit_mult  SystemSampleTime=-1
  reinterp : xbsIndex_r4/Reinterpret  force_arith_type=on  arith_type=Unsigned  force_bin_pt=on  bin_pt=0  block_type=reinterpret
      settings: infoedit="Changes signal type without altering the binary representation.   You can changed the signal between signed and unsigned, and relocate the binary point.<br><br>Hardware notes: In hardware this block costs nothing.<br><br>Example:  Suppose the input is 6 bits wide, signed, with 2 fractional bits, and the output is forced to unsigned with 0 fractional bits.  Then an input of -2.0 (1110.00 in binary 2's complement) becomes an output of 56 (111000 in binary)."
  i-1_out : Outport
  i0_out : Outport  Port=2
  i1_out : Outport  Port=3
  i2_out : Outport  Port=4
  q0_out : Outport  Port=5
  q1_out : Outport  Port=6
  q2_out : Outport  Port=7
  q3_out : Outport  Port=8
  lag_out : Outport  Port=9
  wires:
  i0/1 -> mult_sp0/1, delay_i0/1
  q0/1 -> mult_sp0/2, delay_q0/1
  i1/1 -> mult_sp1/1, delay_i1/1
  q1/1 -> mult_sp1/2, delay_q1/1
  i2/1 -> mult_sp2/1, delay_i2/1
  q2/1 -> mult_sp2/2, delay_q2/1
  i3/1 -> mult_sp3/1, delay_i3/1
  q3/1 -> mult_sp3/2, delay_q3/1
  mult_sp0/1 -> add2/1
  mult_sp1/1 -> add2/2
  mult_sp2/1 -> add1/1
  mult_sp3/1 -> add1/2
  add2/1 -> add0/1
  add1/1 -> add0/2
  delay_i0/1 -> i0_out/1
  delay_q0/1 -> q0_out/1
  delay_i1/1 -> i1_out/1
  delay_q1/1 -> q1_out/1
  delay_i2/1 -> i2_out/1
  delay_q2/1 -> q2_out/1
  delay_i3/1 -> i-1_out/1
  delay_q3/1 -> q3_out/1
  lag_in/1 -> lag_cat/1
  add0/1 -> reinterp/1
  reinterp/1 -> lag_cat/2
  lag_cat/1 -> lag_out/1
